simulink model "Observer"  (Simulink 8.2)
settings: Solver=FixedStepDiscrete  SolverMode=SingleTasking  StartTime=0.0  StopTime=3  FixedStep=Ts  RelTol=1e-3
PreLoadFcn:
  | Ts=1e-3;
libraries: dspbuff3 x1, dspsrcs4 x1
settings Model: Creator=Carchesion  LastModifiedBy=Ugo Pattacini
settings DataIOCC: LimitDataPoints=off  SaveOutput=off  SignalLogging=off  SaveTime=off
settings OptimizationCC: InitFltsAndDblsToZero=on
settings SFSimCC: SimParseCustomCode=off

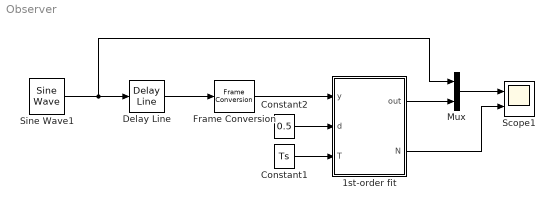
== system Observer ==
  1st-order fit : MATLAB Function  TreatAsAtomicUnit=on
  Constant1 : Constant  Value=Ts
  Constant2 : Constant  Value=0.5
  Delay Line : dspbuff3/Delay Line  siz=16  ic=0  directfeed=off  enable_output=off  hold_output=off  TreatMby1Signals=M channels (this choice will be removed - see release notes)
  Frame Conversion : FrameConversion  OutFrame=Sample-based
  Mux : Mux  Inputs=2
  Scope1 : Scope  NumInputPorts=2
      settings: TimeRange=10  YMin=-5~-5  YMax=5~5
  Sine Wave1 : dspsrcs4/Sine Wave  Amplitude=10  Frequency=1  Phase=0  SampleMode=Discrete  OutComplex=Real  CompMethod=Trigonometric fcn  TableSize=Speed  SampleTime=Ts  SamplesPerFrame=1  ResetState=Restart at time zero  dataType=double  wordLen=16  udDataType=sfix(16)  fracBitsMode=Best precision  numFracBits=15  OutDataTypeStr=double  LastOutDataTypeStr=double
  wires:
  Delay Line/1 -> Frame Conversion/1
  Constant1/1 -> 1st-order fit/3(T)
  Constant2/1 -> 1st-order fit/2(d)
  Frame Conversion/1 -> 1st-order fit/1(y)
  Mux/1 -> Scope1/1
  1st-order fit/2(N) -> Scope1/2
  1st-order fit/1(out) -> Mux/2
  Sine Wave1/1 -> Mux/1, Delay Line/1

== matlab function 1st-order fit ==
  data: y input double; out output double; d input double; T input double; N output double
function [out,N]=fcn(y,d,T)
%#ok<*NASGU>

coder.extrinsic('polyfitHelper');

persistent n;
if isempty(n)
    n=1;
end

L=length(y);
pos=zeros(1,2);
Ly=0;
N=n;

for j=max(1,n-1):min(n+1,L-1)
    pos=polyfitHelper(y,1,T,j);

    finish=false;
    for i=0:j
        Ly=polyval(pos,i*T);
        if abs(y(L-j+i)-Ly)>d
            finish=true;
            break;
        end
    end
    
    if finish
        N=j;
        break;
    end
    N=j;
end

out=pos(1);
n=N;
